simulink model "walkingRobotRL3D"  (R2020b)
settings: Solver=ode23t  StartTime=0.0  StopTime=Tf  RelTol=1e-2  EnableMultiTasking=on
PreLoadFcn:
  | robotParametersRL
undefined symbols (not defined in the file): agent, ankleD_pitch_jointMAX, ankleD_pitch_jointMIN, ankleD_roll_jointMAX, ankleD_roll_jointMIN, ankleI_pitch_jointMAX, ankleI_pitch_jointMIN, ankleI_roll_jointMAX, ankleI_roll_jointMIN, getSampleTime, height_plane, hipD_pitch_jointMAX, hipD_pitch_jointMIN, hipD_roll_jointMAX, hipD_roll_jointMIN, hipI_pitch_jointMAX, hipI_pitch_jointMIN, hipI_roll_jointMAX, hipI_roll_jointMIN, init_angs_L, init_angs_R, init_height, joint_damping, joint_limit_damping, joint_limit_stiffness, joint_stiffness, kneeD_jointMAX, kneeD_jointMIN, kneeI_jointMAX, kneeI_jointMIN, lower_leg_I0, lower_leg_length, lower_leg_mass, lower_leg_x, lower_leg_y, muscle_nominal_length, p10_ankleD_roll, plane_x, plane_y, regulator_type, tau, Tf, torso_height, torso_length, torso_offset_x, torso_offset_z, torso_width, torso_x, torso_y, torso_z, Ts, upper_leg_I0, upper_leg_length, upper_leg_mass, upper_leg_x, upper_leg_y, v10_ankleD_pitch, v10_ankleD_roll, v10_ankleI_pitch, v10_ankleI_roll ... (+41)
libraries: sm_lib x222, simulink x183, nesl_utility x130, walkingRobotUtils x69, rllib x2
(part 16 of 24)

== system walkingRobotRL3D/Walking Robot/DYNAMIC MODEL OF PAM FOR RIGHT LEG/Dynamic Model Antagonisitic PAM1/Spring and damping model/Dynamics muscle 1 ==
  F1 : Inport
  S1 : Inport  Port=2
  R2 : Inport  Port=3
  D1 : Inport  Port=4
  Add : Sum  Inputs=+--
  Add1 : Sum  Inputs=+--
  Constant1 : Constant
  Divide : Product  Inputs=*/
  Integrator : Integrator  InitialCondition=x10_ankleD_pitch
  Unit Delay : UnitDelay  Commented=through  SampleTime=-1  HasFrameUpgradeWarning=on
  Unit Delay1 : UnitDelay  Commented=through  SampleTime=-1  HasFrameUpgradeWarning=on
  Unit Delay2 : UnitDelay  Commented=through  SampleTime=-1  HasFrameUpgradeWarning=on
  x./D1 : Product
  xS1 : Product
  R1 : Outport
  x1 : Outport  Port=2
  wires:
  Integrator/1 -> xS1/1, x1/1
  Divide/1 -> x./D1/1
  F1/1 -> Unit Delay1/1, Add/1
  x./D1/1 -> Integrator/1
  Add/1 -> Unit Delay/1, x./D1/2
  S1/1 -> xS1/2
  Constant1/1 -> Divide/1
  R2/1 -> Add/2
  Unit Delay/1 -> Add1/3
  Add1/1 -> R1/1
  xS1/1 -> Unit Delay2/1, Add/3
  D1/1 -> Divide/2
  Unit Delay1/1 -> Add1/1
  Unit Delay2/1 -> Add1/2

== system walkingRobotRL3D/Walking Robot/DYNAMIC MODEL OF PAM FOR RIGHT LEG/Dynamic Model Antagonisitic PAM2/Spring and damping model/Dynamic muscle 2 ==
  S2 : Inport
  R1 : Inport  Port=2
  F2 : Inport  Port=3
  D2 : Inport  Port=4
  Add : Sum  Inputs=+--
  Add1 : Sum  Inputs=+--
  Constant3 : Constant
  Divide1 : Product  Inputs=*/
  Integrator1 : Integrator  InitialCondition=x20_kneeD
  Unit Delay : UnitDelay  Commented=through  SampleTime=-1  HasFrameUpgradeWarning=on
  Unit Delay1 : UnitDelay  Commented=through  SampleTime=-1  HasFrameUpgradeWarning=on
  Unit Delay2 : UnitDelay  Commented=through  SampleTime=-1  HasFrameUpgradeWarning=on
  x./D2 : Product
  xS2 : Product
  R2 : Outport
  x2 : Outport  Port=2
  wires:
  F2/1 -> Unit Delay1/1, Add1/1
  Divide1/1 -> x./D2/1
  Integrator1/1 -> x2/1, xS2/1
  x./D2/1 -> Integrator1/1
  Add1/1 -> Unit Delay/1, x./D2/2
  Constant3/1 -> Divide1/1
  R1/1 -> Add1/2
  S2/1 -> xS2/2
  Add/1 -> R2/1
  Unit Delay/1 -> Add/3
  xS2/1 -> Unit Delay2/1, Add1/3
  Unit Delay1/1 -> Add/1
  Unit Delay2/1 -> Add/2
  D2/1 -> Divide1/2

== system walkingRobotRL3D/Walking Robot/DYNAMIC MODEL OF PAM FOR RIGHT LEG/Dynamic Model Antagonisitic PAM2/Spring and damping model/Dynamics muscle 1 ==
  F1 : Inport
  S1 : Inport  Port=2
  R2 : Inport  Port=3
  D1 : Inport  Port=4
  Add : Sum  Inputs=+--
  Add1 : Sum  Inputs=+--
  Constant1 : Constant
  Divide : Product  Inputs=*/
  Integrator : Integrator  InitialCondition=x10_kneeD
  Unit Delay : UnitDelay  Commented=through  SampleTime=-1  HasFrameUpgradeWarning=on
  Unit Delay1 : UnitDelay  Commented=through  SampleTime=-1  HasFrameUpgradeWarning=on
  Unit Delay2 : UnitDelay  Commented=through  SampleTime=-1  HasFrameUpgradeWarning=on
  x./D1 : Product
  xS1 : Product
  R1 : Outport
  x1 : Outport  Port=2
  wires:
  Integrator/1 -> xS1/1, x1/1
  Divide/1 -> x./D1/1
  F1/1 -> Unit Delay1/1, Add/1
  x./D1/1 -> Integrator/1
  Add/1 -> Unit Delay/1, x./D1/2
  S1/1 -> xS1/2
  Constant1/1 -> Divide/1
  R2/1 -> Add/2
  Unit Delay/1 -> Add1/3
  Add1/1 -> R1/1
  xS1/1 -> Unit Delay2/1, Add/3
  D1/1 -> Divide/2
  Unit Delay1/1 -> Add1/1
  Unit Delay2/1 -> Add1/2

== system walkingRobotRL3D/Walking Robot/DYNAMIC MODEL OF PAM FOR RIGHT LEG/Dynamic Model Antagonisitic PAM3/Spring and damping model/Dynamic muscle 2 ==
  S2 : Inport
  R1 : Inport  Port=2
  F2 : Inport  Port=3
  D2 : Inport  Port=4
  Add : Sum  Inputs=+--
  Add1 : Sum  Inputs=+--
  Constant3 : Constant
  Divide1 : Product  Inputs=*/
  Integrator1 : Integrator  InitialCondition=x20_ankleD_roll
  Unit Delay : UnitDelay  Commented=through  SampleTime=-1  HasFrameUpgradeWarning=on
  Unit Delay1 : UnitDelay  Commented=through  SampleTime=-1  HasFrameUpgradeWarning=on
  Unit Delay2 : UnitDelay  Commented=through  SampleTime=-1  HasFrameUpgradeWarning=on
  x./D2 : Product
  xS2 : Product
  R2 : Outport
  x2 : Outport  Port=2
  wires:
  F2/1 -> Unit Delay1/1, Add1/1
  Divide1/1 -> x./D2/1
  Integrator1/1 -> x2/1, xS2/1
  x./D2/1 -> Integrator1/1
  Add1/1 -> Unit Delay/1, x./D2/2
  Constant3/1 -> Divide1/1
  R1/1 -> Add1/2
  S2/1 -> xS2/2
  Add/1 -> R2/1
  Unit Delay/1 -> Add/3
  xS2/1 -> Unit Delay2/1, Add1/3
  Unit Delay1/1 -> Add/1
  Unit Delay2/1 -> Add/2
  D2/1 -> Divide1/2

== system walkingRobotRL3D/Walking Robot/DYNAMIC MODEL OF PAM FOR RIGHT LEG/Dynamic Model Antagonisitic PAM3/Spring and damping model/Dynamics muscle 1 ==
  F1 : Inport
  S1 : Inport  Port=2
  R2 : Inport  Port=3
  D1 : Inport  Port=4
  Add : Sum  Inputs=+--
  Add1 : Sum  Inputs=+--
  Constant1 : Constant
  Divide : Product  Inputs=*/
  Integrator : Integrator  InitialCondition=x10_ankleD_roll
  Unit Delay : UnitDelay  Commented=through  SampleTime=-1  HasFrameUpgradeWarning=on
  Unit Delay1 : UnitDelay  Commented=through  SampleTime=-1  HasFrameUpgradeWarning=on
  Unit Delay2 : UnitDelay  Commented=through  SampleTime=-1  HasFrameUpgradeWarning=on
  x./D1 : Product
  xS1 : Product
  R1 : Outport
  x1 : Outport  Port=2
  wires:
  Integrator/1 -> xS1/1, x1/1
  Divide/1 -> x./D1/1
  F1/1 -> Unit Delay1/1, Add/1
  x./D1/1 -> Integrator/1
  Add/1 -> Unit Delay/1, x./D1/2
  S1/1 -> xS1/2
  Constant1/1 -> Divide/1
  R2/1 -> Add/2
  Unit Delay/1 -> Add1/3
  Add1/1 -> R1/1
  xS1/1 -> Unit Delay2/1, Add/3
  D1/1 -> Divide/2
  Unit Delay1/1 -> Add1/1
  Unit Delay2/1 -> Add1/2

== system walkingRobotRL3D/Walking Robot/DYNAMIC MODEL OF PAM FOR RIGHT LEG/Dynamic Model Antagonisitic PAM4/Spring and damping model/Dynamic muscle 2 ==
  S2 : Inport
  R1 : Inport  Port=2
  F2 : Inport  Port=3
  D2 : Inport  Port=4
  Add : Sum  Inputs=+--
  Add1 : Sum  Inputs=+--
  Constant3 : Constant
  Divide1 : Product  Inputs=*/
  Integrator1 : Integrator  InitialCondition=x20_hipD_roll
  Unit Delay : UnitDelay  Commented=through  SampleTime=-1  HasFrameUpgradeWarning=on
  Unit Delay1 : UnitDelay  Commented=through  SampleTime=-1  HasFrameUpgradeWarning=on
  Unit Delay2 : UnitDelay  Commented=through  SampleTime=-1  HasFrameUpgradeWarning=on
  x./D2 : Product
  xS2 : Product
  R2 : Outport
  x2 : Outport  Port=2
  wires:
  F2/1 -> Unit Delay1/1, Add1/1
  Divide1/1 -> x./D2/1
  Integrator1/1 -> x2/1, xS2/1
  x./D2/1 -> Integrator1/1
  Add1/1 -> Unit Delay/1, x./D2/2
  Constant3/1 -> Divide1/1
  R1/1 -> Add1/2
  S2/1 -> xS2/2
  Add/1 -> R2/1
  Unit Delay/1 -> Add/3
  xS2/1 -> Unit Delay2/1, Add1/3
  Unit Delay1/1 -> Add/1
  Unit Delay2/1 -> Add/2
  D2/1 -> Divide1/2

== system walkingRobotRL3D/Walking Robot/DYNAMIC MODEL OF PAM FOR RIGHT LEG/Dynamic Model Antagonisitic PAM4/Spring and damping model/Dynamics muscle 1 ==
  F1 : Inport
  S1 : Inport  Port=2
  R2 : Inport  Port=3
  D1 : Inport  Port=4
  Add : Sum  Inputs=+--
  Add1 : Sum  Inputs=+--
  Constant1 : Constant
  Divide : Product  Inputs=*/
  Integrator : Integrator  InitialCondition=x10_hipD_roll
  Unit Delay : UnitDelay  Commented=through  SampleTime=-1  HasFrameUpgradeWarning=on
  Unit Delay1 : UnitDelay  Commented=through  SampleTime=-1  HasFrameUpgradeWarning=on
  Unit Delay2 : UnitDelay  Commented=through  SampleTime=-1  HasFrameUpgradeWarning=on
  x./D1 : Product
  xS1 : Product
  R1 : Outport
  x1 : Outport  Port=2
  wires:
  Integrator/1 -> xS1/1, x1/1
  Divide/1 -> x./D1/1
  F1/1 -> Unit Delay1/1, Add/1
  x./D1/1 -> Integrator/1
  Add/1 -> Unit Delay/1, x./D1/2
  S1/1 -> xS1/2
  Constant1/1 -> Divide/1
  R2/1 -> Add/2
  Unit Delay/1 -> Add1/3
  Add1/1 -> R1/1
  xS1/1 -> Unit Delay2/1, Add/3
  D1/1 -> Divide/2
  Unit Delay1/1 -> Add1/1
  Unit Delay2/1 -> Add1/2

== system walkingRobotRL3D/Walking Robot/DYNAMIC MODEL OF PAM FOR RIGHT LEG/Dynamic Model Antagonisitic PAM5/Spring and damping model/Dynamic muscle 2 ==
  S2 : Inport
  R1 : Inport  Port=2
  F2 : Inport  Port=3
  D2 : Inport  Port=4
  Add : Sum  Inputs=+--
  Add1 : Sum  Inputs=+--
  Constant3 : Constant
  Divide1 : Product  Inputs=*/
  Integrator1 : Integrator  InitialCondition=x20_hipD_pitch
  Unit Delay : UnitDelay  Commented=through  SampleTime=-1  HasFrameUpgradeWarning=on
  Unit Delay1 : UnitDelay  Commented=through  SampleTime=-1  HasFrameUpgradeWarning=on
  Unit Delay2 : UnitDelay  Commented=through  SampleTime=-1  HasFrameUpgradeWarning=on
  x./D2 : Product
  xS2 : Product
  R2 : Outport
  x2 : Outport  Port=2
  wires:
  F2/1 -> Unit Delay1/1, Add1/1
  Divide1/1 -> x./D2/1
  Integrator1/1 -> x2/1, xS2/1
  x./D2/1 -> Integrator1/1
  Add1/1 -> Unit Delay/1, x./D2/2
  Constant3/1 -> Divide1/1
  R1/1 -> Add1/2
  S2/1 -> xS2/2
  Add/1 -> R2/1
  Unit Delay/1 -> Add/3
  xS2/1 -> Unit Delay2/1, Add1/3
  Unit Delay1/1 -> Add/1
  Unit Delay2/1 -> Add/2
  D2/1 -> Divide1/2

== system walkingRobotRL3D/Walking Robot/DYNAMIC MODEL OF PAM FOR RIGHT LEG/Dynamic Model Antagonisitic PAM5/Spring and damping model/Dynamics muscle 1 ==
  F1 : Inport
  S1 : Inport  Port=2
  R2 : Inport  Port=3
  D1 : Inport  Port=4
  Add : Sum  Inputs=+--
  Add1 : Sum  Inputs=+--
  Constant1 : Constant
  Divide : Product  Inputs=*/
  Integrator : Integrator  InitialCondition=x10_hipD_pitch
  Unit Delay : UnitDelay  Commented=through  SampleTime=-1  HasFrameUpgradeWarning=on
  Unit Delay1 : UnitDelay  Commented=through  SampleTime=-1  HasFrameUpgradeWarning=on
  Unit Delay2 : UnitDelay  Commented=through  SampleTime=-1  HasFrameUpgradeWarning=on
  x./D1 : Product
  xS1 : Product
  R1 : Outport
  x1 : Outport  Port=2
  wires:
  Integrator/1 -> xS1/1, x1/1
  Divide/1 -> x./D1/1
  F1/1 -> Unit Delay1/1, Add/1
  x./D1/1 -> Integrator/1
  Add/1 -> Unit Delay/1, x./D1/2
  S1/1 -> xS1/2
  Constant1/1 -> Divide/1
  R2/1 -> Add/2
  Unit Delay/1 -> Add1/3
  Add1/1 -> R1/1
  xS1/1 -> Unit Delay2/1, Add/3
  D1/1 -> Divide/2
  Unit Delay1/1 -> Add1/1
  Unit Delay2/1 -> Add1/2

== system walkingRobotRL3D/Walking Robot (Angle based)/Antagonistic PAM Left Leg/ankleI_pitch PAM/Spring and damping model/Dynamic muscle 2 ==
  S2 : Inport
  R1 : Inport  Port=2
  F2 : Inport  Port=3
  Add : Sum  Inputs=+--
  Add1 : Sum  Inputs=+--
  Constant2 : Constant  Value=tau
  Constant3 : Constant
  D2dx2 : Scope
  D_coef1 : Product
  Divide1 : Product  Inputs=*/
  Integrator1 : Integrator  InitialCondition=x20_ankleI_pitch
  S2x2 : Scope
  Unit Delay : UnitDelay  SampleTime=-1  HasFrameUpgradeWarning=on
  x./D2 : Product
  xS2 : Product
  R2 : Outport
  x2 : Outport  Port=2
  wires:
  F2/1 -> Add/1, Add1/1
  Divide1/1 -> x./D2/1
  Constant2/1 -> D_coef1/1
  Integrator1/1 -> x2/1, xS2/1
  x./D2/1 -> Integrator1/1
  D_coef1/1 -> Divide1/2
  Add1/1 -> Unit Delay/1, D2dx2/1, x./D2/2
  Constant3/1 -> Divide1/1
  R1/1 -> Add1/2
  S2/1 -> xS2/2, D_coef1/2
  Add/1 -> R2/1
  Unit Delay/1 -> Add/3
  xS2/1 -> S2x2/1, Add/2, Add1/3

== system walkingRobotRL3D/Walking Robot (Angle based)/Antagonistic PAM Left Leg/ankleI_pitch PAM/Spring and damping model/Dynamics muscle 1 ==
  F1 : Inport
  S1 : Inport  Port=2
  R2 : Inport  Port=3
  Add : Sum  Inputs=+--
  Add1 : Sum  Inputs=+--
  Constant : Constant  Value=tau
  Constant1 : Constant
  D1dx1 : Scope
  D_coef : Product
  Divide : Product  Inputs=*/
  Integrator : Integrator  InitialCondition=x10_ankleI_pitch
  S1x1 : Scope
  Unit Delay : UnitDelay  SampleTime=-1  HasFrameUpgradeWarning=on
  x./D1 : Product
  xS1 : Product
  R1 : Outport
  x1 : Outport  Port=2
  wires:
  Constant/1 -> D_coef/1
  Integrator/1 -> xS1/1, x1/1
  Divide/1 -> x./D1/1
  F1/1 -> Add1/1, Add/1
  x./D1/1 -> Integrator/1
  Add/1 -> D1dx1/1, Unit Delay/1, x./D1/2
  S1/1 -> xS1/2, D_coef/2
  Constant1/1 -> Divide/1
  D_coef/1 -> Divide/2
  R2/1 -> Add/2
  Unit Delay/1 -> Add1/3
  Add1/1 -> R1/1
  xS1/1 -> S1x1/1, Add1/2, Add/3

== system walkingRobotRL3D/Walking Robot (Angle based)/Antagonistic PAM Left Leg/ankleI_pitch PAM/Spring and damping model/getDeltaXmax ==
  In1 : Inport
  getMaxStroke1 : MATLAB Function  TreatAsAtomicUnit=on
  dmax1 : Outport
  wires:
  In1/1 -> getMaxStroke1/1(P1)
  getMaxStroke1/1(x_max1) -> dmax1/1

== system walkingRobotRL3D/Walking Robot (Angle based)/Antagonistic PAM Left Leg/ankleI_pitch PAM/Spring and damping model/getDeltaXmax1 ==
  In1 : Inport
  getMaxStroke1 : MATLAB Function  TreatAsAtomicUnit=on
  dmax2 : Outport
  wires:
  In1/1 -> getMaxStroke1/1(P2)
  getMaxStroke1/1(x_max1) -> dmax2/1

== system walkingRobotRL3D/Walking Robot (Angle based)/Antagonistic PAM Left Leg/ankleI_roll PAM/Spring and damping model/Dynamic muscle 2 ==
  S2 : Inport
  R1 : Inport  Port=2
  F2 : Inport  Port=3
  Add : Sum  Inputs=+--
  Add1 : Sum  Inputs=+--
  Constant2 : Constant  Value=tau
  Constant3 : Constant
  D2dx2 : Scope
  D_coef1 : Product
  Divide1 : Product  Inputs=*/
  Integrator1 : Integrator  InitialCondition=x20_ankleI_roll
  S2x2 : Scope
  Unit Delay : UnitDelay  SampleTime=-1  HasFrameUpgradeWarning=on
  x./D2 : Product
  xS2 : Product
  R2 : Outport
  x2 : Outport  Port=2
  wires:
  F2/1 -> Add/1, Add1/1
  Divide1/1 -> x./D2/1
  Constant2/1 -> D_coef1/1
  Integrator1/1 -> x2/1, xS2/1
  x./D2/1 -> Integrator1/1
  D_coef1/1 -> Divide1/2
  Add1/1 -> Unit Delay/1, D2dx2/1, x./D2/2
  Constant3/1 -> Divide1/1
  R1/1 -> Add1/2
  S2/1 -> xS2/2, D_coef1/2
  Add/1 -> R2/1
  Unit Delay/1 -> Add/3
  xS2/1 -> S2x2/1, Add/2, Add1/3

== system walkingRobotRL3D/Walking Robot (Angle based)/Antagonistic PAM Left Leg/ankleI_roll PAM/Spring and damping model/Dynamics muscle 1 ==
  F1 : Inport
  S1 : Inport  Port=2
  R2 : Inport  Port=3
  Add : Sum  Inputs=+--
  Add1 : Sum  Inputs=+--
  Constant : Constant  Value=tau
  Constant1 : Constant
  D1dx1 : Scope
  D_coef : Product
  Divide : Product  Inputs=*/
  Integrator : Integrator  InitialCondition=x10_ankleI_roll
  S1x1 : Scope
  Unit Delay : UnitDelay  SampleTime=-1  HasFrameUpgradeWarning=on
  x./D1 : Product
  xS1 : Product
  R1 : Outport
  x1 : Outport  Port=2
  wires:
  Constant/1 -> D_coef/1
  Integrator/1 -> xS1/1, x1/1
  Divide/1 -> x./D1/1
  F1/1 -> Add1/1, Add/1
  x./D1/1 -> Integrator/1
  Add/1 -> D1dx1/1, Unit Delay/1, x./D1/2
  S1/1 -> xS1/2, D_coef/2
  Constant1/1 -> Divide/1
  D_coef/1 -> Divide/2
  R2/1 -> Add/2
  Unit Delay/1 -> Add1/3
  Add1/1 -> R1/1
  xS1/1 -> S1x1/1, Add1/2, Add/3

== system walkingRobotRL3D/Walking Robot (Angle based)/Antagonistic PAM Left Leg/ankleI_roll PAM/Spring and damping model/getDeltaXmax ==
  In1 : Inport
  getMaxStroke1 : MATLAB Function  TreatAsAtomicUnit=on
  dmax1 : Outport
  wires:
  In1/1 -> getMaxStroke1/1(P1)
  getMaxStroke1/1(x_max1) -> dmax1/1

== system walkingRobotRL3D/Walking Robot (Angle based)/Antagonistic PAM Left Leg/ankleI_roll PAM/Spring and damping model/getDeltaXmax1 ==
  In1 : Inport
  getMaxStroke1 : MATLAB Function  TreatAsAtomicUnit=on
  dmax2 : Outport
  wires:
  In1/1 -> getMaxStroke1/1(P2)
  getMaxStroke1/1(x_max1) -> dmax2/1

== system walkingRobotRL3D/Walking Robot (Angle based)/Antagonistic PAM Left Leg/hipI_pitch PAM/Spring and damping model/Dynamic muscle 2 ==
  S2 : Inport
  R1 : Inport  Port=2
  F2 : Inport  Port=3
  Add : Sum  Inputs=+--
  Add1 : Sum  Inputs=+--
  Constant2 : Constant  Value=tau
  Constant3 : Constant
  D2dx2 : Scope
  D_coef1 : Product
  Divide1 : Product  Inputs=*/
  Integrator1 : Integrator  InitialCondition=x20_hipI_pitch
  S2x2 : Scope
  Unit Delay : UnitDelay  SampleTime=-1  HasFrameUpgradeWarning=on
  x./D2 : Product
  xS2 : Product
  R2 : Outport
  x2 : Outport  Port=2
  wires:
  F2/1 -> Add/1, Add1/1
  Divide1/1 -> x./D2/1
  Constant2/1 -> D_coef1/1
  Integrator1/1 -> x2/1, xS2/1
  x./D2/1 -> Integrator1/1
  D_coef1/1 -> Divide1/2
  Add1/1 -> Unit Delay/1, D2dx2/1, x./D2/2
  Constant3/1 -> Divide1/1
  R1/1 -> Add1/2
  S2/1 -> xS2/2, D_coef1/2
  Add/1 -> R2/1
  Unit Delay/1 -> Add/3
  xS2/1 -> S2x2/1, Add/2, Add1/3

== system walkingRobotRL3D/Walking Robot (Angle based)/Antagonistic PAM Left Leg/hipI_pitch PAM/Spring and damping model/Dynamics muscle 1 ==
  F1 : Inport
  S1 : Inport  Port=2
  R2 : Inport  Port=3
  Add : Sum  Inputs=+--
  Add1 : Sum  Inputs=+--
  Constant : Constant  Value=tau
  Constant1 : Constant
  D1dx1 : Scope
  D_coef : Product
  Divide : Product  Inputs=*/
  Integrator : Integrator  InitialCondition=x10_hipI_pitch
  S1x1 : Scope
  Unit Delay : UnitDelay  SampleTime=-1  HasFrameUpgradeWarning=on
  x./D1 : Product
  xS1 : Product
  R1 : Outport
  x1 : Outport  Port=2
  wires:
  Constant/1 -> D_coef/1
  Integrator/1 -> xS1/1, x1/1
  Divide/1 -> x./D1/1
  F1/1 -> Add1/1, Add/1
  x./D1/1 -> Integrator/1
  Add/1 -> D1dx1/1, Unit Delay/1, x./D1/2
  S1/1 -> xS1/2, D_coef/2
  Constant1/1 -> Divide/1
  D_coef/1 -> Divide/2
  R2/1 -> Add/2
  Unit Delay/1 -> Add1/3
  Add1/1 -> R1/1
  xS1/1 -> S1x1/1, Add1/2, Add/3

== system walkingRobotRL3D/Walking Robot (Angle based)/Antagonistic PAM Left Leg/hipI_pitch PAM/Spring and damping model/getDeltaXmax ==
  In1 : Inport
  getMaxStroke1 : MATLAB Function  TreatAsAtomicUnit=on
  dmax1 : Outport
  wires:
  In1/1 -> getMaxStroke1/1(P1)
  getMaxStroke1/1(x_max1) -> dmax1/1

== system walkingRobotRL3D/Walking Robot (Angle based)/Antagonistic PAM Left Leg/hipI_pitch PAM/Spring and damping model/getDeltaXmax1 ==
  In1 : Inport
  getMaxStroke1 : MATLAB Function  TreatAsAtomicUnit=on
  dmax2 : Outport
  wires:
  In1/1 -> getMaxStroke1/1(P2)
  getMaxStroke1/1(x_max1) -> dmax2/1

== system walkingRobotRL3D/Walking Robot (Angle based)/Antagonistic PAM Left Leg/hipI_roll PAM/Spring and damping model/Dynamic muscle 2 ==
  S2 : Inport
  R1 : Inport  Port=2
  F2 : Inport  Port=3
  Add : Sum  Inputs=+--
  Add1 : Sum  Inputs=+--
  Constant2 : Constant  Value=tau
  Constant3 : Constant
  D2dx2 : Scope
  D_coef1 : Product
  Divide1 : Product  Inputs=*/
  Integrator1 : Integrator  InitialCondition=x20_hipI_roll
  S2x2 : Scope
  Unit Delay : UnitDelay  SampleTime=-1  HasFrameUpgradeWarning=on
  x./D2 : Product
  xS2 : Product
  R2 : Outport
  x2 : Outport  Port=2
  wires:
  F2/1 -> Add/1, Add1/1
  Divide1/1 -> x./D2/1
  Constant2/1 -> D_coef1/1
  Integrator1/1 -> x2/1, xS2/1
  x./D2/1 -> Integrator1/1
  D_coef1/1 -> Divide1/2
  Add1/1 -> Unit Delay/1, D2dx2/1, x./D2/2
  Constant3/1 -> Divide1/1
  R1/1 -> Add1/2
  S2/1 -> xS2/2, D_coef1/2
  Add/1 -> R2/1
  Unit Delay/1 -> Add/3
  xS2/1 -> S2x2/1, Add/2, Add1/3

== system walkingRobotRL3D/Walking Robot (Angle based)/Antagonistic PAM Left Leg/hipI_roll PAM/Spring and damping model/Dynamics muscle 1 ==
  F1 : Inport
  S1 : Inport  Port=2
  R2 : Inport  Port=3
  Add : Sum  Inputs=+--
  Add1 : Sum  Inputs=+--
  Constant : Constant  Value=tau
  Constant1 : Constant
  D1dx1 : Scope
  D_coef : Product
  Divide : Product  Inputs=*/
  Integrator : Integrator  InitialCondition=x10_hipI_roll
  S1x1 : Scope
  Unit Delay : UnitDelay  SampleTime=-1  HasFrameUpgradeWarning=on
  x./D1 : Product
  xS1 : Product
  R1 : Outport
  x1 : Outport  Port=2
  wires:
  Constant/1 -> D_coef/1
  Integrator/1 -> xS1/1, x1/1
  Divide/1 -> x./D1/1
  F1/1 -> Add1/1, Add/1
  x./D1/1 -> Integrator/1
  Add/1 -> D1dx1/1, Unit Delay/1, x./D1/2
  S1/1 -> xS1/2, D_coef/2
  Constant1/1 -> Divide/1
  D_coef/1 -> Divide/2
  R2/1 -> Add/2
  Unit Delay/1 -> Add1/3
  Add1/1 -> R1/1
  xS1/1 -> S1x1/1, Add1/2, Add/3

== system walkingRobotRL3D/Walking Robot (Angle based)/Antagonistic PAM Left Leg/hipI_roll PAM/Spring and damping model/getDeltaXmax ==
  In1 : Inport
  getMaxStroke1 : MATLAB Function  TreatAsAtomicUnit=on
  dmax1 : Outport
  wires:
  In1/1 -> getMaxStroke1/1(P1)
  getMaxStroke1/1(x_max1) -> dmax1/1

== system walkingRobotRL3D/Walking Robot (Angle based)/Antagonistic PAM Left Leg/hipI_roll PAM/Spring and damping model/getDeltaXmax1 ==
  In1 : Inport
  getMaxStroke1 : MATLAB Function  TreatAsAtomicUnit=on
  dmax2 : Outport
  wires:
  In1/1 -> getMaxStroke1/1(P2)
  getMaxStroke1/1(x_max1) -> dmax2/1

== system walkingRobotRL3D/Walking Robot (Angle based)/Antagonistic PAM Left Leg/kneeI PAM/Spring and damping model/Dynamic muscle 2 ==
  S2 : Inport
  R1 : Inport  Port=2
  F2 : Inport  Port=3
  Add : Sum  Inputs=+--
  Add1 : Sum  Inputs=+--
  Constant2 : Constant  Value=tau
  Constant3 : Constant
  D2dx2 : Scope
  D_coef1 : Product
  Divide1 : Product  Inputs=*/
  Integrator1 : Integrator  InitialCondition=x20_kneeI
  S2x2 : Scope
  Unit Delay : UnitDelay  SampleTime=-1  HasFrameUpgradeWarning=on
  x./D2 : Product
  xS2 : Product
  R2 : Outport
  x2 : Outport  Port=2
  wires:
  F2/1 -> Add/1, Add1/1
  Divide1/1 -> x./D2/1
  Constant2/1 -> D_coef1/1
  Integrator1/1 -> x2/1, xS2/1
  x./D2/1 -> Integrator1/1
  D_coef1/1 -> Divide1/2
  Add1/1 -> Unit Delay/1, D2dx2/1, x./D2/2
  Constant3/1 -> Divide1/1
  R1/1 -> Add1/2
  S2/1 -> xS2/2, D_coef1/2
  Add/1 -> R2/1
  Unit Delay/1 -> Add/3
  xS2/1 -> S2x2/1, Add/2, Add1/3

== system walkingRobotRL3D/Walking Robot (Angle based)/Antagonistic PAM Left Leg/kneeI PAM/Spring and damping model/Dynamics muscle 1 ==
  F1 : Inport
  S1 : Inport  Port=2
  R2 : Inport  Port=3
  Add : Sum  Inputs=+--
  Add1 : Sum  Inputs=+--
  Constant : Constant  Value=tau
  Constant1 : Constant
  D1dx1 : Scope
  D_coef : Product
  Divide : Product  Inputs=*/
  Integrator : Integrator  InitialCondition=x10_kneeI
  S1x1 : Scope
  Unit Delay : UnitDelay  SampleTime=-1  HasFrameUpgradeWarning=on
  x./D1 : Product
  xS1 : Product
  R1 : Outport
  x1 : Outport  Port=2
  wires:
  Constant/1 -> D_coef/1
  Integrator/1 -> xS1/1, x1/1
  Divide/1 -> x./D1/1
  F1/1 -> Add1/1, Add/1
  x./D1/1 -> Integrator/1
  Add/1 -> D1dx1/1, Unit Delay/1, x./D1/2
  S1/1 -> xS1/2, D_coef/2
  Constant1/1 -> Divide/1
  D_coef/1 -> Divide/2
  R2/1 -> Add/2
  Unit Delay/1 -> Add1/3
  Add1/1 -> R1/1
  xS1/1 -> S1x1/1, Add1/2, Add/3

== system walkingRobotRL3D/Walking Robot (Angle based)/Antagonistic PAM Left Leg/kneeI PAM/Spring and damping model/getDeltaXmax ==
  In1 : Inport
  getMaxStroke1 : MATLAB Function  TreatAsAtomicUnit=on
  dmax1 : Outport
  wires:
  In1/1 -> getMaxStroke1/1(P1)
  getMaxStroke1/1(x_max1) -> dmax1/1

== system walkingRobotRL3D/Walking Robot (Angle based)/Antagonistic PAM Left Leg/kneeI PAM/Spring and damping model/getDeltaXmax1 ==
  In1 : Inport
  getMaxStroke1 : MATLAB Function  TreatAsAtomicUnit=on
  dmax2 : Outport
  wires:
  In1/1 -> getMaxStroke1/1(P2)
  getMaxStroke1/1(x_max1) -> dmax2/1

== system walkingRobotRL3D/Walking Robot (Angle based)/Antagonistic PAM Right Leg/ankleD_pitch PAM/Spring and damping model/Dynamic muscle 2 ==
  S2 : Inport
  R1 : Inport  Port=2
  F2 : Inport  Port=3
  Add : Sum  Inputs=+--
  Add1 : Sum  Inputs=+--
  Constant2 : Constant  Value=tau
  Constant3 : Constant
  D2dx2 : Scope
  D_coef1 : Product
  Divide1 : Product  Inputs=*/
  Integrator1 : Integrator  InitialCondition=x20_ankleD_pitch
  S2x2 : Scope
  Unit Delay : UnitDelay  SampleTime=-1  HasFrameUpgradeWarning=on
  x./D2 : Product
  xS2 : Product
  R2 : Outport
  x2 : Outport  Port=2
  wires:
  F2/1 -> Add/1, Add1/1
  Divide1/1 -> x./D2/1
  Constant2/1 -> D_coef1/1
  Integrator1/1 -> x2/1, xS2/1
  x./D2/1 -> Integrator1/1
  D_coef1/1 -> Divide1/2
  Add1/1 -> Unit Delay/1, D2dx2/1, x./D2/2
  Constant3/1 -> Divide1/1
  R1/1 -> Add1/2
  S2/1 -> xS2/2, D_coef1/2
  Add/1 -> R2/1
  Unit Delay/1 -> Add/3
  xS2/1 -> S2x2/1, Add/2, Add1/3

== system walkingRobotRL3D/Walking Robot (Angle based)/Antagonistic PAM Right Leg/ankleD_pitch PAM/Spring and damping model/Dynamics muscle 1 ==
  F1 : Inport
  S1 : Inport  Port=2
  R2 : Inport  Port=3
  Add : Sum  Inputs=+--
  Add1 : Sum  Inputs=+--
  Constant : Constant  Value=tau
  Constant1 : Constant
  D1dx1 : Scope
  D_coef : Product
  Divide : Product  Inputs=*/
  Integrator : Integrator  InitialCondition=x10_ankleD_pitch
  S1x1 : Scope
  Unit Delay : UnitDelay  SampleTime=-1  HasFrameUpgradeWarning=on
  x./D1 : Product
  xS1 : Product
  R1 : Outport
  x1 : Outport  Port=2
  wires:
  Constant/1 -> D_coef/1
  Integrator/1 -> xS1/1, x1/1
  Divide/1 -> x./D1/1
  F1/1 -> Add1/1, Add/1
  x./D1/1 -> Integrator/1
  Add/1 -> D1dx1/1, Unit Delay/1, x./D1/2
  S1/1 -> xS1/2, D_coef/2
  Constant1/1 -> Divide/1
  D_coef/1 -> Divide/2
  R2/1 -> Add/2
  Unit Delay/1 -> Add1/3
  Add1/1 -> R1/1
  xS1/1 -> S1x1/1, Add1/2, Add/3

== system walkingRobotRL3D/Walking Robot (Angle based)/Antagonistic PAM Right Leg/ankleD_pitch PAM/Spring and damping model/getDeltaXmax ==
  In1 : Inport
  getMaxStroke1 : MATLAB Function  TreatAsAtomicUnit=on
  dmax1 : Outport
  wires:
  In1/1 -> getMaxStroke1/1(P1)
  getMaxStroke1/1(x_max1) -> dmax1/1

== system walkingRobotRL3D/Walking Robot (Angle based)/Antagonistic PAM Right Leg/ankleD_pitch PAM/Spring and damping model/getDeltaXmax1 ==
  In1 : Inport
  getMaxStroke1 : MATLAB Function  TreatAsAtomicUnit=on
  dmax2 : Outport
  wires:
  In1/1 -> getMaxStroke1/1(P2)
  getMaxStroke1/1(x_max1) -> dmax2/1

== system walkingRobotRL3D/Walking Robot (Angle based)/Antagonistic PAM Right Leg/ankleD_roll PAM/Spring and damping model/Dynamic muscle 2 ==
  S2 : Inport
  R1 : Inport  Port=2
  F2 : Inport  Port=3
  Add : Sum  Inputs=+--
  Add1 : Sum  Inputs=+--
  Constant2 : Constant  Value=tau
  Constant3 : Constant
  D2dx2 : Scope
  D_coef1 : Product
  Divide1 : Product  Inputs=*/
  Integrator1 : Integrator  InitialCondition=x20_ankleD_roll
  S2x2 : Scope
  Unit Delay : UnitDelay  SampleTime=-1  HasFrameUpgradeWarning=on
  x./D2 : Product
  xS2 : Product
  R2 : Outport
  x2 : Outport  Port=2
  wires:
  F2/1 -> Add/1, Add1/1
  Divide1/1 -> x./D2/1
  Constant2/1 -> D_coef1/1
  Integrator1/1 -> x2/1, xS2/1
  x./D2/1 -> Integrator1/1
  D_coef1/1 -> Divide1/2
  Add1/1 -> Unit Delay/1, D2dx2/1, x./D2/2
  Constant3/1 -> Divide1/1
  R1/1 -> Add1/2
  S2/1 -> xS2/2, D_coef1/2
  Add/1 -> R2/1
  Unit Delay/1 -> Add/3
  xS2/1 -> S2x2/1, Add/2, Add1/3

== system walkingRobotRL3D/Walking Robot (Angle based)/Antagonistic PAM Right Leg/ankleD_roll PAM/Spring and damping model/Dynamics muscle 1 ==
  F1 : Inport
  S1 : Inport  Port=2
  R2 : Inport  Port=3
  Add : Sum  Inputs=+--
  Add1 : Sum  Inputs=+--
  Constant : Constant  Value=tau
  Constant1 : Constant
  D1dx1 : Scope
  D_coef : Product
  Divide : Product  Inputs=*/
  Integrator : Integrator  InitialCondition=x10_ankleD_roll
  S1x1 : Scope
  Unit Delay : UnitDelay  SampleTime=-1  HasFrameUpgradeWarning=on
  x./D1 : Product
  xS1 : Product
  R1 : Outport
  x1 : Outport  Port=2
  wires:
  Constant/1 -> D_coef/1
  Integrator/1 -> xS1/1, x1/1
  Divide/1 -> x./D1/1
  F1/1 -> Add1/1, Add/1
  x./D1/1 -> Integrator/1
  Add/1 -> D1dx1/1, Unit Delay/1, x./D1/2
  S1/1 -> xS1/2, D_coef/2
  Constant1/1 -> Divide/1
  D_coef/1 -> Divide/2
  R2/1 -> Add/2
  Unit Delay/1 -> Add1/3
  Add1/1 -> R1/1
  xS1/1 -> S1x1/1, Add1/2, Add/3

== system walkingRobotRL3D/Walking Robot (Angle based)/Antagonistic PAM Right Leg/ankleD_roll PAM/Spring and damping model/getDeltaXmax ==
  In1 : Inport
  getMaxStroke1 : MATLAB Function  TreatAsAtomicUnit=on
  dmax1 : Outport
  wires:
  In1/1 -> getMaxStroke1/1(P1)
  getMaxStroke1/1(x_max1) -> dmax1/1

== system walkingRobotRL3D/Walking Robot (Angle based)/Antagonistic PAM Right Leg/ankleD_roll PAM/Spring and damping model/getDeltaXmax1 ==
  In1 : Inport
  getMaxStroke1 : MATLAB Function  TreatAsAtomicUnit=on
  dmax2 : Outport
  wires:
  In1/1 -> getMaxStroke1/1(P2)
  getMaxStroke1/1(x_max1) -> dmax2/1

== system walkingRobotRL3D/Walking Robot (Angle based)/Antagonistic PAM Right Leg/hipD_pitch PAM/Spring and damping model/Dynamic muscle 2 ==
  S2 : Inport
  R1 : Inport  Port=2
  F2 : Inport  Port=3
  Add : Sum  Inputs=+--
  Add1 : Sum  Inputs=+--
  Constant2 : Constant  Value=tau
  Constant3 : Constant
  D2dx2 : Scope
  D_coef1 : Product
  Divide1 : Product  Inputs=*/
  Integrator1 : Integrator  InitialCondition=x20_hipD_pitch
  S2x2 : Scope
  Unit Delay : UnitDelay  SampleTime=-1  HasFrameUpgradeWarning=on
  x./D2 : Product
  xS2 : Product
  R2 : Outport
  x2 : Outport  Port=2
  wires:
  F2/1 -> Add/1, Add1/1
  Divide1/1 -> x./D2/1
  Constant2/1 -> D_coef1/1
  Integrator1/1 -> x2/1, xS2/1
  x./D2/1 -> Integrator1/1
  D_coef1/1 -> Divide1/2
  Add1/1 -> Unit Delay/1, D2dx2/1, x./D2/2
  Constant3/1 -> Divide1/1
  R1/1 -> Add1/2
  S2/1 -> xS2/2, D_coef1/2
  Add/1 -> R2/1
  Unit Delay/1 -> Add/3
  xS2/1 -> S2x2/1, Add/2, Add1/3

== system walkingRobotRL3D/Walking Robot (Angle based)/Antagonistic PAM Right Leg/hipD_pitch PAM/Spring and damping model/Dynamics muscle 1 ==
  F1 : Inport
  S1 : Inport  Port=2
  R2 : Inport  Port=3
  Add : Sum  Inputs=+--
  Add1 : Sum  Inputs=+--
  Constant : Constant  Value=tau
  Constant1 : Constant
  D1dx1 : Scope
  D_coef : Product
  Divide : Product  Inputs=*/
  Integrator : Integrator  InitialCondition=x10_hipD_pitch
  S1x1 : Scope
  Unit Delay : UnitDelay  SampleTime=-1  HasFrameUpgradeWarning=on
  x./D1 : Product
  xS1 : Product
  R1 : Outport
  x1 : Outport  Port=2
  wires:
  Constant/1 -> D_coef/1
  Integrator/1 -> xS1/1, x1/1
  Divide/1 -> x./D1/1
  F1/1 -> Add1/1, Add/1
  x./D1/1 -> Integrator/1
  Add/1 -> D1dx1/1, Unit Delay/1, x./D1/2
  S1/1 -> xS1/2, D_coef/2
  Constant1/1 -> Divide/1
  D_coef/1 -> Divide/2
  R2/1 -> Add/2
  Unit Delay/1 -> Add1/3
  Add1/1 -> R1/1
  xS1/1 -> S1x1/1, Add1/2, Add/3

== system walkingRobotRL3D/Walking Robot (Angle based)/Antagonistic PAM Right Leg/hipD_pitch PAM/Spring and damping model/getDeltaXmax ==
  In1 : Inport
  getMaxStroke1 : MATLAB Function  TreatAsAtomicUnit=on
  dmax1 : Outport
  wires:
  In1/1 -> getMaxStroke1/1(P1)
  getMaxStroke1/1(x_max1) -> dmax1/1

== system walkingRobotRL3D/Walking Robot (Angle based)/Antagonistic PAM Right Leg/hipD_pitch PAM/Spring and damping model/getDeltaXmax1 ==
  In1 : Inport
  getMaxStroke1 : MATLAB Function  TreatAsAtomicUnit=on
  dmax2 : Outport
  wires:
  In1/1 -> getMaxStroke1/1(P2)
  getMaxStroke1/1(x_max1) -> dmax2/1

== system walkingRobotRL3D/Walking Robot (Angle based)/Antagonistic PAM Right Leg/hipD_roll PAM/Spring and damping model/Dynamic muscle 2 ==
  S2 : Inport
  R1 : Inport  Port=2
  F2 : Inport  Port=3
  Add : Sum  Inputs=+--
  Add1 : Sum  Inputs=+--
  Constant2 : Constant  Value=tau
  Constant3 : Constant
  D2dx2 : Scope
  D_coef1 : Product
  Divide1 : Product  Inputs=*/
  Integrator1 : Integrator  InitialCondition=x20_hipD_roll
  S2x2 : Scope
  Unit Delay : UnitDelay  SampleTime=-1  HasFrameUpgradeWarning=on
  x./D2 : Product
  xS2 : Product
  R2 : Outport
  x2 : Outport  Port=2
  wires:
  F2/1 -> Add/1, Add1/1
  Divide1/1 -> x./D2/1
  Constant2/1 -> D_coef1/1
  Integrator1/1 -> x2/1, xS2/1
  x./D2/1 -> Integrator1/1
  D_coef1/1 -> Divide1/2
  Add1/1 -> Unit Delay/1, D2dx2/1, x./D2/2
  Constant3/1 -> Divide1/1
  R1/1 -> Add1/2
  S2/1 -> xS2/2, D_coef1/2
  Add/1 -> R2/1
  Unit Delay/1 -> Add/3
  xS2/1 -> S2x2/1, Add/2, Add1/3

== system walkingRobotRL3D/Walking Robot (Angle based)/Antagonistic PAM Right Leg/hipD_roll PAM/Spring and damping model/Dynamics muscle 1 ==
  F1 : Inport
  S1 : Inport  Port=2
  R2 : Inport  Port=3
  Add : Sum  Inputs=+--
  Add1 : Sum  Inputs=+--
  Constant : Constant  Value=tau
  Constant1 : Constant
  D1dx1 : Scope
  D_coef : Product
  Divide : Product  Inputs=*/
  Integrator : Integrator  InitialCondition=x10_hipD_roll
  S1x1 : Scope
  Unit Delay : UnitDelay  SampleTime=-1  HasFrameUpgradeWarning=on
  x./D1 : Product
  xS1 : Product
  R1 : Outport
  x1 : Outport  Port=2
  wires:
  Constant/1 -> D_coef/1
  Integrator/1 -> xS1/1, x1/1
  Divide/1 -> x./D1/1
  F1/1 -> Add1/1, Add/1
  x./D1/1 -> Integrator/1
  Add/1 -> D1dx1/1, Unit Delay/1, x./D1/2
  S1/1 -> xS1/2, D_coef/2
  Constant1/1 -> Divide/1
  D_coef/1 -> Divide/2
  R2/1 -> Add/2
  Unit Delay/1 -> Add1/3
  Add1/1 -> R1/1
  xS1/1 -> S1x1/1, Add1/2, Add/3

== system walkingRobotRL3D/Walking Robot (Angle based)/Antagonistic PAM Right Leg/hipD_roll PAM/Spring and damping model/getDeltaXmax ==
  In1 : Inport
  getMaxStroke1 : MATLAB Function  TreatAsAtomicUnit=on
  dmax1 : Outport
  wires:
  In1/1 -> getMaxStroke1/1(P1)
  getMaxStroke1/1(x_max1) -> dmax1/1

== system walkingRobotRL3D/Walking Robot (Angle based)/Antagonistic PAM Right Leg/hipD_roll PAM/Spring and damping model/getDeltaXmax1 ==
  In1 : Inport
  getMaxStroke1 : MATLAB Function  TreatAsAtomicUnit=on
  dmax2 : Outport
  wires:
  In1/1 -> getMaxStroke1/1(P2)
  getMaxStroke1/1(x_max1) -> dmax2/1

== system walkingRobotRL3D/Walking Robot (Angle based)/Antagonistic PAM Right Leg/kneeD PAM/Spring and damping model/Dynamic muscle 2 ==
  S2 : Inport
  R1 : Inport  Port=2
  F2 : Inport  Port=3
  Add : Sum  Inputs=+--
  Add1 : Sum  Inputs=+--
  Constant2 : Constant  Value=tau
  Constant3 : Constant
  D2dx2 : Scope
  D_coef1 : Product
  Divide1 : Product  Inputs=*/
  Integrator1 : Integrator  InitialCondition=x20_kneeD
  S2x2 : Scope
  Unit Delay : UnitDelay  SampleTime=-1  HasFrameUpgradeWarning=on
  x./D2 : Product
  xS2 : Product
  R2 : Outport
  x2 : Outport  Port=2
  wires:
  F2/1 -> Add/1, Add1/1
  Divide1/1 -> x./D2/1
  Constant2/1 -> D_coef1/1
  Integrator1/1 -> x2/1, xS2/1
  x./D2/1 -> Integrator1/1
  D_coef1/1 -> Divide1/2
  Add1/1 -> Unit Delay/1, D2dx2/1, x./D2/2
  Constant3/1 -> Divide1/1
  R1/1 -> Add1/2
  S2/1 -> xS2/2, D_coef1/2
  Add/1 -> R2/1
  Unit Delay/1 -> Add/3
  xS2/1 -> S2x2/1, Add/2, Add1/3

== system walkingRobotRL3D/Walking Robot (Angle based)/Antagonistic PAM Right Leg/kneeD PAM/Spring and damping model/Dynamics muscle 1 ==
  F1 : Inport
  S1 : Inport  Port=2
  R2 : Inport  Port=3
  Add : Sum  Inputs=+--
  Add1 : Sum  Inputs=+--
  Constant : Constant  Value=tau
  Constant1 : Constant
  D1dx1 : Scope
  D_coef : Product
  Divide : Product  Inputs=*/
  Integrator : Integrator  InitialCondition=x10_kneeD
  S1x1 : Scope
  Unit Delay : UnitDelay  SampleTime=-1  HasFrameUpgradeWarning=on
  x./D1 : Product
  xS1 : Product
  R1 : Outport
  x1 : Outport  Port=2
  wires:
  Constant/1 -> D_coef/1
  Integrator/1 -> xS1/1, x1/1
  Divide/1 -> x./D1/1
  F1/1 -> Add1/1, Add/1
  x./D1/1 -> Integrator/1
  Add/1 -> D1dx1/1, Unit Delay/1, x./D1/2
  S1/1 -> xS1/2, D_coef/2
  Constant1/1 -> Divide/1
  D_coef/1 -> Divide/2
  R2/1 -> Add/2
  Unit Delay/1 -> Add1/3
  Add1/1 -> R1/1
  xS1/1 -> S1x1/1, Add1/2, Add/3

== system walkingRobotRL3D/Walking Robot (Angle based)/Antagonistic PAM Right Leg/kneeD PAM/Spring and damping model/getDeltaXmax ==
  In1 : Inport
  getMaxStroke1 : MATLAB Function  TreatAsAtomicUnit=on
  dmax1 : Outport
  wires:
  In1/1 -> getMaxStroke1/1(P1)
  getMaxStroke1/1(x_max1) -> dmax1/1

== system walkingRobotRL3D/Walking Robot (Angle based)/Antagonistic PAM Right Leg/kneeD PAM/Spring and damping model/getDeltaXmax1 ==
  In1 : Inport
  getMaxStroke1 : MATLAB Function  TreatAsAtomicUnit=on
  dmax2 : Outport
  wires:
  In1/1 -> getMaxStroke1/1(P2)
  getMaxStroke1/1(x_max1) -> dmax2/1

== system walkingRobotRL3D/Walking Robot (Angle based)/Dynamic model of antagonistic PAM actuators/Spring//Damping (Muscles 1)/Get_delta_xmax1/getDeltaXmax ==
  In1 : Inport
  Delay4 : Delay  DelayLength=1  InitialCondition=x10_ankleD_roll*100/muscle_nominal_length
  Delay5 : Delay  DelayLength=1  InitialCondition=0
  MATLAB Function : MATLAB Function  TreatAsAtomicUnit=on
  Subsystem : Subsystem  Commented=on
  Subtract3 : Sum  Inputs=+-
  getMaxStroke1 : MATLAB Function  TreatAsAtomicUnit=on
  Out1 : Outport
  Out2 : Outport  Port=2
  wires:
  In1/1 -> getMaxStroke1/1(P1)
  getMaxStroke1/1(x_max1) -> Delay4/1, Subtract3/1, MATLAB Function/1(x)
  Delay4/1 -> MATLAB Function/2(xant)
  MATLAB Function/1(savex) -> Out2/1, Subtract3/2, Delay5/1
  Delay5/1 -> MATLAB Function/3(save)
  Subtract3/1 -> Out1/1

== system walkingRobotRL3D/Walking Robot (Angle based)/Dynamic model of antagonistic PAM actuators/Spring//Damping (Muscles 1)/Get_delta_xmax1/getDeltaXmax1 ==
  In1 : Inport
  Delay4 : Delay  DelayLength=1  InitialCondition=x10_ankleD_pitch*100/muscle_nominal_length
  Delay5 : Delay  DelayLength=1  InitialCondition=0
  MATLAB Function : MATLAB Function  TreatAsAtomicUnit=on
  Subtract3 : Sum  Inputs=+-
  getMaxStroke1 : MATLAB Function  TreatAsAtomicUnit=on
  Out1 : Outport
  Out2 : Outport  Port=2
  wires:
  In1/1 -> getMaxStroke1/1(P1)
  getMaxStroke1/1(x_max1) -> Delay4/1, Subtract3/1, MATLAB Function/1(x)
  Delay4/1 -> MATLAB Function/2(xant)
  MATLAB Function/1(savex) -> Out2/1, Subtract3/2, Delay5/1
  Delay5/1 -> MATLAB Function/3(save)
  Subtract3/1 -> Out1/1

== system walkingRobotRL3D/Walking Robot (Angle based)/Dynamic model of antagonistic PAM actuators/Spring//Damping (Muscles 1)/Get_delta_xmax1/getDeltaXmax2 ==
  In1 : Inport
  Delay4 : Delay  DelayLength=1  InitialCondition=x10_kneeD*100/muscle_nominal_length
  Delay5 : Delay  DelayLength=1  InitialCondition=0
  MATLAB Function : MATLAB Function  TreatAsAtomicUnit=on
  Subtract3 : Sum  Inputs=+-
  getMaxStroke1 : MATLAB Function  TreatAsAtomicUnit=on
  Out1 : Outport
  Out2 : Outport  Port=2
  wires:
  In1/1 -> getMaxStroke1/1(P1)
  getMaxStroke1/1(x_max1) -> Delay4/1, Subtract3/1, MATLAB Function/1(x)
  Delay4/1 -> MATLAB Function/2(xant)
  MATLAB Function/1(savex) -> Out2/1, Subtract3/2, Delay5/1
  Delay5/1 -> MATLAB Function/3(save)
  Subtract3/1 -> Out1/1

== system walkingRobotRL3D/Walking Robot (Angle based)/Dynamic model of antagonistic PAM actuators/Spring//Damping (Muscles 1)/Get_delta_xmax1/getDeltaXmax3 ==
  In1 : Inport
  Delay4 : Delay  DelayLength=1  InitialCondition=x10_hipD_roll*100/muscle_nominal_length
  Delay5 : Delay  DelayLength=1  InitialCondition=0
  MATLAB Function : MATLAB Function  TreatAsAtomicUnit=on
  Subtract3 : Sum  Inputs=+-
  getMaxStroke1 : MATLAB Function  TreatAsAtomicUnit=on
  Out1 : Outport
  Out2 : Outport  Port=2
  wires:
  In1/1 -> getMaxStroke1/1(P1)
  getMaxStroke1/1(x_max1) -> Delay4/1, Subtract3/1, MATLAB Function/1(x)
  Delay4/1 -> MATLAB Function/2(xant)
  MATLAB Function/1(savex) -> Out2/1, Subtract3/2, Delay5/1
  Delay5/1 -> MATLAB Function/3(save)
  Subtract3/1 -> Out1/1

== system walkingRobotRL3D/Walking Robot (Angle based)/Dynamic model of antagonistic PAM actuators/Spring//Damping (Muscles 1)/Get_delta_xmax1/getDeltaXmax4 ==
  In1 : Inport
  Delay4 : Delay  DelayLength=1  InitialCondition=x10_hipD_pitch*100/muscle_nominal_length
  Delay5 : Delay  DelayLength=1  InitialCondition=0
  MATLAB Function : MATLAB Function  TreatAsAtomicUnit=on
  Subtract3 : Sum  Inputs=+-
  getMaxStroke1 : MATLAB Function  TreatAsAtomicUnit=on
  Out1 : Outport
  Out2 : Outport  Port=2
  wires:
  In1/1 -> getMaxStroke1/1(P1)
  getMaxStroke1/1(x_max1) -> Delay4/1, Subtract3/1, MATLAB Function/1(x)
  Delay4/1 -> MATLAB Function/2(xant)
  MATLAB Function/1(savex) -> Out2/1, Subtract3/2, Delay5/1
  Delay5/1 -> MATLAB Function/3(save)
  Subtract3/1 -> Out1/1

== system walkingRobotRL3D/Walking Robot (Angle based)/Dynamic model of antagonistic PAM actuators/Spring//Damping (Muscles 1)/Get_delta_xmax1/getDeltaXmax5 ==
  In1 : Inport
  Delay4 : Delay  DelayLength=1  InitialCondition=x10_ankleI_roll*100/muscle_nominal_length
  Delay5 : Delay  DelayLength=1  InitialCondition=0
  MATLAB Function : MATLAB Function  TreatAsAtomicUnit=on
  Subtract3 : Sum  Inputs=+-
  getMaxStroke1 : MATLAB Function  TreatAsAtomicUnit=on
  Out1 : Outport
  Out2 : Outport  Port=2
  wires:
  In1/1 -> getMaxStroke1/1(P1)
  getMaxStroke1/1(x_max1) -> Delay4/1, Subtract3/1, MATLAB Function/1(x)
  Delay4/1 -> MATLAB Function/2(xant)
  MATLAB Function/1(savex) -> Out2/1, Subtract3/2, Delay5/1
  Delay5/1 -> MATLAB Function/3(save)
  Subtract3/1 -> Out1/1

== system walkingRobotRL3D/Walking Robot (Angle based)/Dynamic model of antagonistic PAM actuators/Spring//Damping (Muscles 1)/Get_delta_xmax1/getDeltaXmax6 ==
  In1 : Inport
  Delay4 : Delay  DelayLength=1  InitialCondition=x10_ankleI_pitch*100/muscle_nominal_length
  Delay5 : Delay  DelayLength=1  InitialCondition=0
  MATLAB Function : MATLAB Function  TreatAsAtomicUnit=on
  Subtract3 : Sum  Inputs=+-
  getMaxStroke1 : MATLAB Function  TreatAsAtomicUnit=on
  Out1 : Outport
  Out2 : Outport  Port=2
  wires:
  In1/1 -> getMaxStroke1/1(P1)
  getMaxStroke1/1(x_max1) -> Delay4/1, Subtract3/1, MATLAB Function/1(x)
  Delay4/1 -> MATLAB Function/2(xant)
  MATLAB Function/1(savex) -> Out2/1, Subtract3/2, Delay5/1
  Delay5/1 -> MATLAB Function/3(save)
  Subtract3/1 -> Out1/1

== system walkingRobotRL3D/Walking Robot (Angle based)/Dynamic model of antagonistic PAM actuators/Spring//Damping (Muscles 1)/Get_delta_xmax1/getDeltaXmax7 ==
  In1 : Inport
  Delay4 : Delay  DelayLength=1  InitialCondition=x10_kneeI*100/muscle_nominal_length
  Delay5 : Delay  DelayLength=1  InitialCondition=0
  MATLAB Function : MATLAB Function  TreatAsAtomicUnit=on
  Subtract3 : Sum  Inputs=+-
  getMaxStroke1 : MATLAB Function  TreatAsAtomicUnit=on
  Out1 : Outport
  Out2 : Outport  Port=2
  wires:
  In1/1 -> getMaxStroke1/1(P1)
  getMaxStroke1/1(x_max1) -> Delay4/1, Subtract3/1, MATLAB Function/1(x)
  Delay4/1 -> MATLAB Function/2(xant)
  MATLAB Function/1(savex) -> Out2/1, Subtract3/2, Delay5/1
  Delay5/1 -> MATLAB Function/3(save)
  Subtract3/1 -> Out1/1

== system walkingRobotRL3D/Walking Robot (Angle based)/Dynamic model of antagonistic PAM actuators/Spring//Damping (Muscles 1)/Get_delta_xmax1/getDeltaXmax8 ==
  In1 : Inport
  Delay4 : Delay  DelayLength=1  InitialCondition=x10_hipI_roll*100/muscle_nominal_length
  Delay5 : Delay  DelayLength=1  InitialCondition=0
  MATLAB Function : MATLAB Function  TreatAsAtomicUnit=on
  Subtract3 : Sum  Inputs=+-
  getMaxStroke1 : MATLAB Function  TreatAsAtomicUnit=on
  Out1 : Outport
  Out2 : Outport  Port=2
  wires:
  In1/1 -> getMaxStroke1/1(P1)
  getMaxStroke1/1(x_max1) -> Delay4/1, Subtract3/1, MATLAB Function/1(x)
  Delay4/1 -> MATLAB Function/2(xant)
  MATLAB Function/1(savex) -> Out2/1, Subtract3/2, Delay5/1
  Delay5/1 -> MATLAB Function/3(save)
  Subtract3/1 -> Out1/1

== system walkingRobotRL3D/Walking Robot (Angle based)/Dynamic model of antagonistic PAM actuators/Spring//Damping (Muscles 1)/Get_delta_xmax1/getDeltaXmax9 ==
  In1 : Inport
  Delay4 : Delay  DelayLength=1  InitialCondition=x10_hipI_pitch*100/muscle_nominal_length
  Delay5 : Delay  DelayLength=1  InitialCondition=0
  MATLAB Function : MATLAB Function  TreatAsAtomicUnit=on
  Subtract3 : Sum  Inputs=+-
  getMaxStroke1 : MATLAB Function  TreatAsAtomicUnit=on
  Out1 : Outport
  Out2 : Outport  Port=2
  wires:
  In1/1 -> getMaxStroke1/1(P1)
  getMaxStroke1/1(x_max1) -> Delay4/1, Subtract3/1, MATLAB Function/1(x)
  Delay4/1 -> MATLAB Function/2(xant)
  MATLAB Function/1(savex) -> Out2/1, Subtract3/2, Delay5/1
  Delay5/1 -> MATLAB Function/3(save)
  Subtract3/1 -> Out1/1

== system walkingRobotRL3D/Walking Robot (Angle based)/Dynamic model of antagonistic PAM actuators/Spring//Damping (Muscles 2)/Getxmax2/Get_delta_xmax1 ==
  P2 : Inport
  Bar->kPa : Product
  Constant : Constant  Value=100
  Demux : Demux  Outputs=10
  Mux : Mux  Inputs=10
  Mux1 : Mux  Inputs=10
  getDeltaXmax : Subsystem
  getDeltaXmax1 : Subsystem
  getDeltaXmax2 : Subsystem
  getDeltaXmax3 : Subsystem
  getDeltaXmax4 : Subsystem
  getDeltaXmax5 : Subsystem
  getDeltaXmax6 : Subsystem
  getDeltaXmax7 : Subsystem
  getDeltaXmax8 : Subsystem
  getDeltaXmax9 : Subsystem
  delta_xmax_muscles2 : Outport
  delta_xmax_muscles2_per : Outport  Port=2
  wires:
  P2/1 -> Bar->kPa/2
  Bar->kPa/1 -> Demux/1
  Constant/1 -> Bar->kPa/1
  Mux/1 -> delta_xmax_muscles2/1
  Demux/1 -> getDeltaXmax/1(In1)
  getDeltaXmax/1(Out1) -> Mux/1
  Mux1/1 -> delta_xmax_muscles2_per/1
  getDeltaXmax/2(Out2) -> Mux1/1
  Demux/2 -> getDeltaXmax1/1(In1)
  Demux/3 -> getDeltaXmax2/1(In1)
  Demux/4 -> getDeltaXmax3/1(In1)
  Demux/5 -> getDeltaXmax4/1(In1)
  Demux/6 -> getDeltaXmax5/1(In1)
  Demux/7 -> getDeltaXmax6/1(In1)
  Demux/8 -> getDeltaXmax7/1(In1)
  Demux/9 -> getDeltaXmax8/1(In1)
  Demux/10 -> getDeltaXmax9/1(In1)
  getDeltaXmax1/1(Out1) -> Mux/2
  getDeltaXmax2/1(Out1) -> Mux/3
  getDeltaXmax3/1(Out1) -> Mux/4
  getDeltaXmax4/1(Out1) -> Mux/5
  getDeltaXmax5/1(Out1) -> Mux/6
  getDeltaXmax6/1(Out1) -> Mux/7
  getDeltaXmax7/1(Out1) -> Mux/8
  getDeltaXmax8/1(Out1) -> Mux/9
  getDeltaXmax9/1(Out1) -> Mux/10
  getDeltaXmax1/2(Out2) -> Mux1/2
  getDeltaXmax2/2(Out2) -> Mux1/3
  getDeltaXmax3/2(Out2) -> Mux1/4
  getDeltaXmax4/2(Out2) -> Mux1/5
  getDeltaXmax5/2(Out2) -> Mux1/6
  getDeltaXmax6/2(Out2) -> Mux1/7
  getDeltaXmax7/2(Out2) -> Mux1/8
  getDeltaXmax8/2(Out2) -> Mux1/9
  getDeltaXmax9/2(Out2) -> Mux1/10

== system walkingRobotRL3D/Walking Robot33/DYNAMIC MODEL OF PAM FOR LEFT LEG/Dynamic Model Antagonisitic PAM1/Spring and damping model/Dynamic muscle 2 ==
  S2 : Inport
  R1 : Inport  Port=2
  F2 : Inport  Port=3
  D2 : Inport  Port=4
  Add : Sum  Inputs=+--
  Add1 : Sum  Inputs=+--
  Constant3 : Constant
  Divide1 : Product  Inputs=*/
  Integrator1 : Integrator  InitialCondition=x20_ankleI_pitch
  Unit Delay : UnitDelay  Commented=through  SampleTime=-1  HasFrameUpgradeWarning=on
  Unit Delay1 : UnitDelay  Commented=through  SampleTime=-1  HasFrameUpgradeWarning=on
  Unit Delay2 : UnitDelay  Commented=through  SampleTime=-1  HasFrameUpgradeWarning=on
  x./D2 : Product
  xS2 : Product
  R2 : Outport
  x2 : Outport  Port=2
  wires:
  F2/1 -> Unit Delay1/1, Add1/1
  Divide1/1 -> x./D2/1
  Integrator1/1 -> x2/1, xS2/1
  x./D2/1 -> Integrator1/1
  Add1/1 -> Unit Delay/1, x./D2/2
  Constant3/1 -> Divide1/1
  R1/1 -> Add1/2
  S2/1 -> xS2/2
  Add/1 -> R2/1
  Unit Delay/1 -> Add/3
  xS2/1 -> Unit Delay2/1, Add1/3
  Unit Delay1/1 -> Add/1
  Unit Delay2/1 -> Add/2
  D2/1 -> Divide1/2

== system walkingRobotRL3D/Walking Robot33/DYNAMIC MODEL OF PAM FOR LEFT LEG/Dynamic Model Antagonisitic PAM1/Spring and damping model/Dynamics muscle 1 ==
  F1 : Inport
  S1 : Inport  Port=2
  R2 : Inport  Port=3
  D1 : Inport  Port=4
  Add : Sum  Inputs=+--
  Add1 : Sum  Inputs=+--
  Constant1 : Constant
  Divide : Product  Inputs=*/
  Integrator : Integrator  InitialCondition=x10_ankleI_pitch
  Unit Delay : UnitDelay  Commented=through  SampleTime=-1  HasFrameUpgradeWarning=on
  Unit Delay1 : UnitDelay  Commented=through  SampleTime=-1  HasFrameUpgradeWarning=on
  Unit Delay2 : UnitDelay  Commented=through  SampleTime=-1  HasFrameUpgradeWarning=on
  x./D1 : Product
  xS1 : Product
  R1 : Outport
  x1 : Outport  Port=2
  wires:
  Integrator/1 -> xS1/1, x1/1
  Divide/1 -> x./D1/1
  F1/1 -> Unit Delay1/1, Add/1
  x./D1/1 -> Integrator/1
  Add/1 -> Unit Delay/1, x./D1/2
  S1/1 -> xS1/2
  Constant1/1 -> Divide/1
  R2/1 -> Add/2
  Unit Delay/1 -> Add1/3
  Add1/1 -> R1/1
  xS1/1 -> Unit Delay2/1, Add/3
  D1/1 -> Divide/2
  Unit Delay1/1 -> Add1/1
  Unit Delay2/1 -> Add1/2

== system walkingRobotRL3D/Walking Robot33/DYNAMIC MODEL OF PAM FOR LEFT LEG/Dynamic Model Antagonisitic PAM2/Spring and damping model/Dynamic muscle 2 ==
  S2 : Inport
  R1 : Inport  Port=2
  F2 : Inport  Port=3
  D2 : Inport  Port=4
  Add : Sum  Inputs=+--
  Add1 : Sum  Inputs=+--
  Constant3 : Constant
  Divide1 : Product  Inputs=*/
  Integrator1 : Integrator  InitialCondition=x20_kneeI
  Unit Delay : UnitDelay  Commented=through  SampleTime=-1  HasFrameUpgradeWarning=on
  Unit Delay1 : UnitDelay  Commented=through  SampleTime=-1  HasFrameUpgradeWarning=on
  Unit Delay2 : UnitDelay  Commented=through  SampleTime=-1  HasFrameUpgradeWarning=on
  x./D2 : Product
  xS2 : Product
  R2 : Outport
  x2 : Outport  Port=2
  wires:
  F2/1 -> Unit Delay1/1, Add1/1
  Divide1/1 -> x./D2/1
  Integrator1/1 -> x2/1, xS2/1
  x./D2/1 -> Integrator1/1
  Add1/1 -> Unit Delay/1, x./D2/2
  Constant3/1 -> Divide1/1
  R1/1 -> Add1/2
  S2/1 -> xS2/2
  Add/1 -> R2/1
  Unit Delay/1 -> Add/3
  xS2/1 -> Unit Delay2/1, Add1/3
  Unit Delay1/1 -> Add/1
  Unit Delay2/1 -> Add/2
  D2/1 -> Divide1/2

== system walkingRobotRL3D/Walking Robot33/DYNAMIC MODEL OF PAM FOR LEFT LEG/Dynamic Model Antagonisitic PAM2/Spring and damping model/Dynamics muscle 1 ==
  F1 : Inport
  S1 : Inport  Port=2
  R2 : Inport  Port=3
  D1 : Inport  Port=4
  Add : Sum  Inputs=+--
  Add1 : Sum  Inputs=+--
  Constant1 : Constant
  Divide : Product  Inputs=*/
  Integrator : Integrator  InitialCondition=x10_kneeI
  Unit Delay : UnitDelay  Commented=through  SampleTime=-1  HasFrameUpgradeWarning=on
  Unit Delay1 : UnitDelay  Commented=through  SampleTime=-1  HasFrameUpgradeWarning=on
  Unit Delay2 : UnitDelay  Commented=through  SampleTime=-1  HasFrameUpgradeWarning=on
  x./D1 : Product
  xS1 : Product
  R1 : Outport
  x1 : Outport  Port=2
  wires:
  Integrator/1 -> xS1/1, x1/1
  Divide/1 -> x./D1/1
  F1/1 -> Unit Delay1/1, Add/1
  x./D1/1 -> Integrator/1
  Add/1 -> Unit Delay/1, x./D1/2
  S1/1 -> xS1/2
  Constant1/1 -> Divide/1
  R2/1 -> Add/2
  Unit Delay/1 -> Add1/3
  Add1/1 -> R1/1
  xS1/1 -> Unit Delay2/1, Add/3
  D1/1 -> Divide/2
  Unit Delay1/1 -> Add1/1
  Unit Delay2/1 -> Add1/2
